simulink model "B52CostaTest"  (R2022a)
settings: Solver=VariableStepAuto  StartTime=0.0  StopTime=100  RelTol=1e-4  AbsTol=1e-4
values from neighbouring files (symbols this model uses):
  AinfK_h_B52 = -23    [B52.m]
  AinfK_p_B52 = 1.0    (= 1)    [B52.m]
  AinfK_s_B52 = 9.0    (= 9)    [B52.m]
  AinfNa_h_B52 = -37    [B52.m]
  AinfNa_p_B52 = 1.0    (= 1)    [B52.m]
  AinfNa_s_B52 = 5.0    (= 5)    [B52.m]
  AinfNarb_h_B52 = -61    [B52.m]    (also in CtrlParaSNSTuning.m)
  AinfNarb_p_B52 = 3    [B52.m]    (also in CtrlParaSNSTuning.m)
  AinfNarb_s_B52 = -1.0    (= -1)    [B52.m]    (also in CtrlParaSNSTuning.m)
  AK_B52_0 = 0.4    [B52.m]
  ANa_B52_0 = 0.4    [B52.m]
  ANarb_B52_0 = 0.1    [B52.m]    (also in CtrlParaSNSTuning.m; InitPara.m)
  BinfNa_h_B52 = -43.0    (= -43)    [B52.m]
  BinfNa_p_B52 = 1.0    (= 1)    [B52.m]
  BinfNa_s_B52 = 5.0    (= 5)    [B52.m]
  BNa_B52_0 = 0.4    [B52.m]
  Cm_B52 = 0.01    [B52.m]    (also in CtrlParaSNSTuning.m)
  EK_B52 = -70    [B52.m]
  EL_B52 = -62    [B52.m]    (also in CtrlParaSNSTuning.m)
  ENa_B52 = 30    [B52.m]
  ENarb_B52 = 30    [B52.m]    (also in CtrlParaSNSTuning.m)
  gK_B52 = 12    [B52.m]
  gL_B52 = 0.1    [B52.m]    (also in CtrlParaSNSTuning.m)
  gNa_B52 = 25    [B52.m]
  gNarb_B52 = 0.1    [B52.m]    (also in CtrlParaSNSTuning.m)
  pK_B52 = 4    [B52.m]
  pNa_B52 = 3    [B52.m]
  pNarb_B52 = 1    [B52.m]    (also in CtrlParaSNSTuning.m)
  RK_B52 = 0    [B52.m]
  RL_B52 = 0    [B52.m]    (also in CtrlParaSNSTuning.m)
  RNa_B52 = 0    [B52.m]
  RNarb_B52 = 0    [B52.m]    (also in CtrlParaSNSTuning.m)
  spikedur_B52 = 0.003    [B52.m]
  tAK_h_B52 = -8.0    (= -8)    [B52.m]
  tAK_p_B52 = 1.0    (= 1)    [B52.m]
  tAK_s_B52 = 10.0    (= 10)    [B52.m]
  tAK_tmax_B52 = 0.04    [B52.m]
  tAK_tmin_B52 = 0.004    [B52.m]
  tANa_h_B52 = -43    [B52.m]
  tANa_p_B52 = 1.0    (= 1)    [B52.m]
  tANa_s_B52 = 4.0    (= 4)    [B52.m]
  tANa_tmax_B52 = 0.006    [B52.m]
  tANa_tmin_B52 = 0.001    [B52.m]
  tANarb_h_B52 = -60    [B52.m]    (also in CtrlParaSNSTuning.m)
  tANarb_p_B52 = 1.0    (= 1)    [B52.m]    (also in CtrlParaSNSTuning.m)
  tANarb_s_B52 = 5    [B52.m]    (also in CtrlParaSNSTuning.m)
  tANarb_tmax_B52 = 20    [B52.m]    (also in CtrlParaSNSTuning.m)
  tANarb_tmin_B52 = 5    [B52.m]    (also in CtrlParaSNSTuning.m)
  tBNa_h_B52 = -38    [B52.m]
  tBNa_p_B52 = 1.0    (= 1)    [B52.m]
  tBNa_s_B52 = 10.0    (= 10)    [B52.m]
  tBNa_tmax_B52 = 0.02    [B52.m]
  tBNa_tmin_B52 = 0.005    [B52.m]
  V_B52_0 = -60    [B52.m]    (also in CtrlParaSNSTuning.m = -62; InitPara.m = -62)
undefined symbols (not defined in the file or in its folder): Iapp
libraries: simulink x1
settings Model: Creator=liyan  LastModifiedBy=liyan

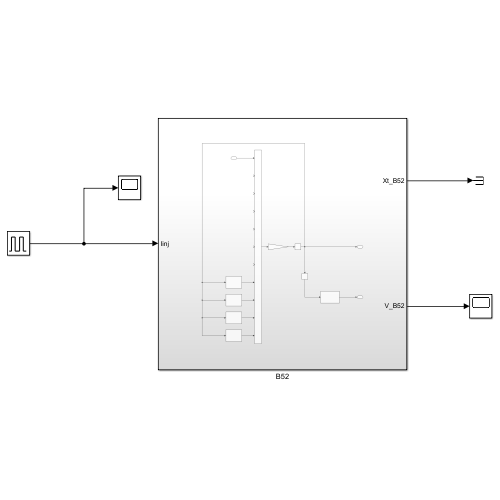
[thumbnail: Simulink's stored preview of the top-level diagram]
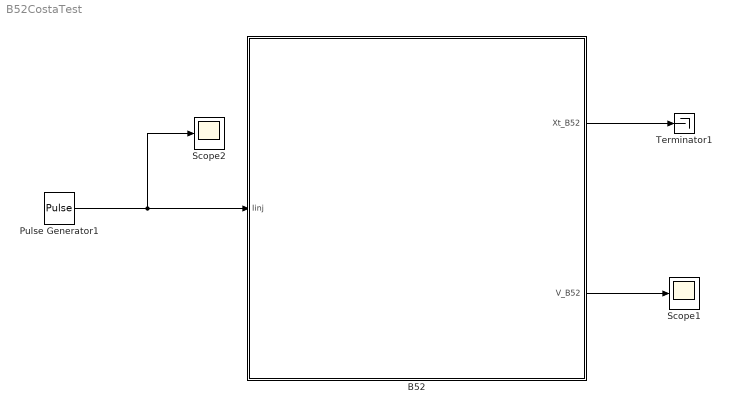
== system B52CostaTest ==
  B52 : Subsystem
  Pulse Generator1 : DiscretePulseGenerator  PulseType=Time based  Amplitude=Iapp  Period=100  PulseWidth=10/100*100  PhaseDelay=35
  Scope1 : Scope
  Scope2 : Scope
  Terminator1 : Terminator
  wires:
  Pulse Generator1/1 -> B52/1(Iinj), Scope2/1
  B52/2(Xt_B52) -> Terminator1/1
  B52/1(V_B52) -> Scope1/1

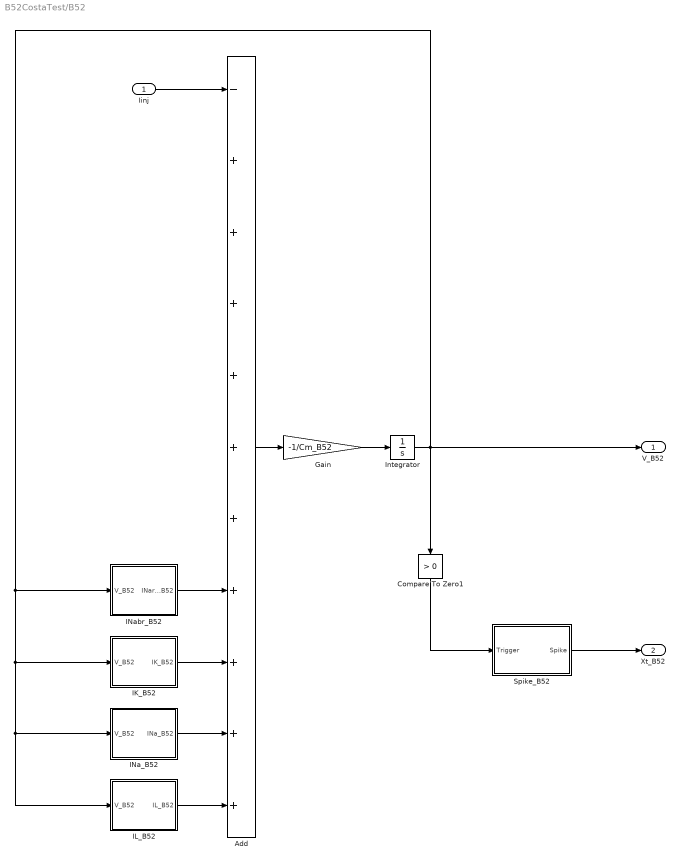
== system B52CostaTest/B52 ==
  Iinj : Inport
  Add : Sum  Inputs=-++++++++++
  Compare To Zero1 : simulink/Logic and Bit Operations/Compare To Zero  relop=>  OutDataTypeStr=boolean
  Gain : Gain  Gain=-1/Cm_B52
  IK_B52 : Subsystem
  IL_B52 : Subsystem
  INa_B52 : Subsystem
  INabr_B52 : Subsystem
  Integrator : Integrator  InitialCondition=V_B52_0
  Spike_B52 : Subsystem
  V_B52 : Outport
  Xt_B52 : Outport  Port=2
  wires:
  Gain/1 -> Integrator/1
  Add/1 -> Gain/1
  Compare To Zero1/1 -> Spike_B52/1(Trigger)
  INabr_B52/1(INarb_B52) -> Add/8
  Spike_B52/1(Spike) -> Xt_B52/1
  Integrator/1 -> V_B52/1, Compare To Zero1/1, INabr_B52/1(V_B52), IK_B52/1(V_B52), INa_B52/1(V_B52), IL_B52/1(V_B52)
  IL_B52/1(IL_B52) -> Add/11
  INa_B52/1(INa_B52) -> Add/10
  IK_B52/1(IK_B52) -> Add/9
  Iinj/1 -> Add/1

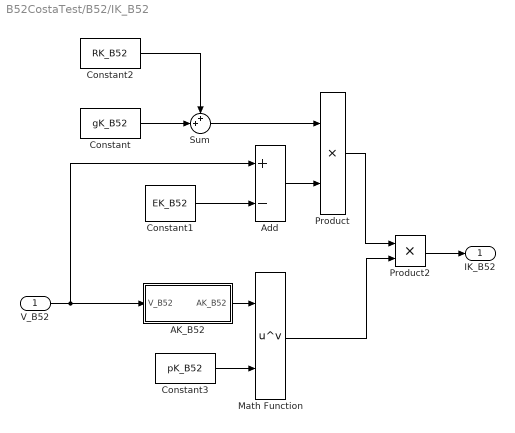
== system B52CostaTest/B52/IK_B52 ==
  V_B52 : Inport
  AK_B52 : Subsystem
  Add : Sum  Inputs=+-
  Constant : Constant  Value=gK_B52
  Constant1 : Constant  Value=EK_B52
  Constant2 : Constant  Value=RK_B52
  Constant3 : Constant  Value=pK_B52
  Math Function : Math  Operator=pow
  Product : Product
  Product2 : Product
  Sum : Sum  Inputs=++|
  IK_B52 : Outport
  wires:
  Add/1 -> Product/2
  Constant1/1 -> Add/2
  V_B52/1 -> AK_B52/1(V_B52), Add/1
  Product/1 -> Product2/1
  Math Function/1 -> Product2/2
  Product2/1 -> IK_B52/1
  Constant/1 -> Sum/2
  Sum/1 -> Product/1
  Constant2/1 -> Sum/1
  AK_B52/1(AK_B52) -> Math Function/1
  Constant3/1 -> Math Function/2

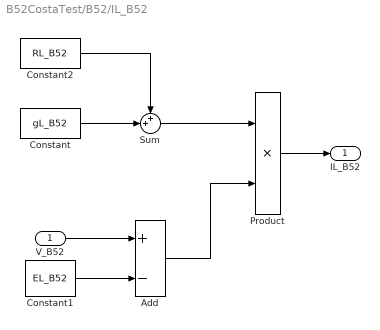
== system B52CostaTest/B52/IL_B52 ==
  V_B52 : Inport
  Add : Sum  Inputs=+-
  Constant : Constant  Value=gL_B52
  Constant1 : Constant  Value=EL_B52
  Constant2 : Constant  Value=RL_B52
  Product : Product
  Sum : Sum  Inputs=++|
  IL_B52 : Outport
  wires:
  Constant1/1 -> Add/2
  V_B52/1 -> Add/1
  Constant2/1 -> Sum/1
  Sum/1 -> Product/1
  Constant/1 -> Sum/2
  Add/1 -> Product/2
  Product/1 -> IL_B52/1

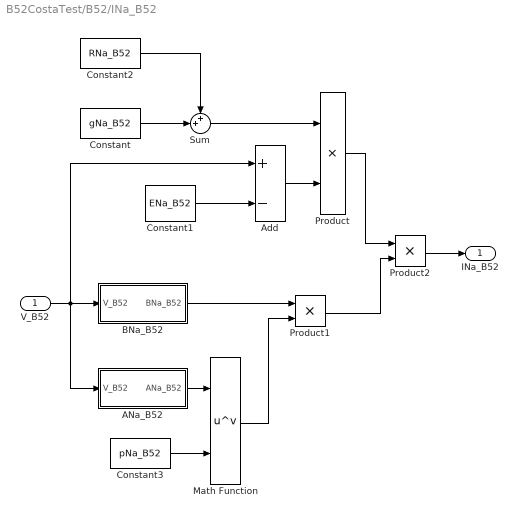
== system B52CostaTest/B52/INa_B52 ==
  V_B52 : Inport
  ANa_B52 : Subsystem
  Add : Sum  Inputs=+-
  BNa_B52 : Subsystem
  Constant : Constant  Value=gNa_B52
  Constant1 : Constant  Value=ENa_B52
  Constant2 : Constant  Value=RNa_B52
  Constant3 : Constant  Value=pNa_B52
  Math Function : Math  Operator=pow
  Product : Product
  Product1 : Product
  Product2 : Product
  Sum : Sum  Inputs=++|
  INa_B52 : Outport
  wires:
  Add/1 -> Product/2
  Constant1/1 -> Add/2
  V_B52/1 -> ANa_B52/1(V_B52), BNa_B52/1(V_B52), Add/1
  Product/1 -> Product2/1
  Product1/1 -> Product2/2
  Product2/1 -> INa_B52/1
  Constant/1 -> Sum/2
  Sum/1 -> Product/1
  Constant2/1 -> Sum/1
  ANa_B52/1(ANa_B52) -> Math Function/1
  Constant3/1 -> Math Function/2
  BNa_B52/1(BNa_B52) -> Product1/1
  Math Function/1 -> Product1/2

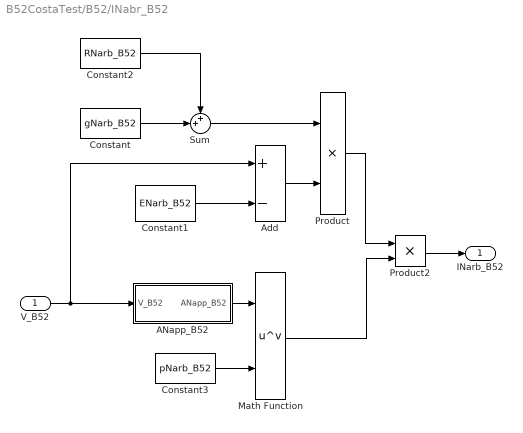
== system B52CostaTest/B52/INabr_B52 ==
  V_B52 : Inport
  ANapp_B52 : Subsystem
  Add : Sum  Inputs=+-
  Constant : Constant  Value=gNarb_B52
  Constant1 : Constant  Value=ENarb_B52
  Constant2 : Constant  Value=RNarb_B52
  Constant3 : Constant  Value=pNarb_B52
  Math Function : Math  Operator=pow
  Product : Product
  Product2 : Product
  Sum : Sum  Inputs=++|
  INarb_B52 : Outport
  wires:
  Add/1 -> Product/2
  Constant1/1 -> Add/2
  V_B52/1 -> ANapp_B52/1(V_B52), Add/1
  Product/1 -> Product2/1
  Math Function/1 -> Product2/2
  Product2/1 -> INarb_B52/1
  Constant/1 -> Sum/2
  Sum/1 -> Product/1
  Constant2/1 -> Sum/1
  ANapp_B52/1(ANapp_B52) -> Math Function/1
  Constant3/1 -> Math Function/2

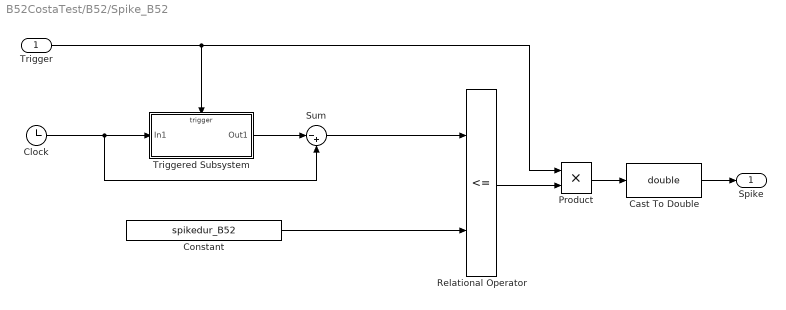
== system B52CostaTest/B52/Spike_B52 ==
  Trigger : Inport
  Cast To Double : DataTypeConversion  OutDataTypeStr=double  SaturateOnIntegerOverflow=off  RndMeth=Floor
  Clock : Clock
  Constant : Constant  Value=spikedur_B52
  Product : Product
  Relational Operator : RelationalOperator  Operator=<=  OutDataTypeStr=boolean  RndMeth=Simplest  InputSameDT=off
  Sum : Sum  Inputs=|-+
  Triggered Subsystem : Subsystem  TreatAsAtomicUnit=on
  Spike : Outport
  wires:
  Clock/1 -> Sum/2, Triggered Subsystem/1(In1)
  Triggered Subsystem/1(Out1) -> Sum/1
  Constant/1 -> Relational Operator/2
  Trigger/1 -> Triggered Subsystem/Trigger, Product/1
  Sum/1 -> Relational Operator/1
  Relational Operator/1 -> Product/2
  Product/1 -> Cast To Double/1
  Cast To Double/1 -> Spike/1

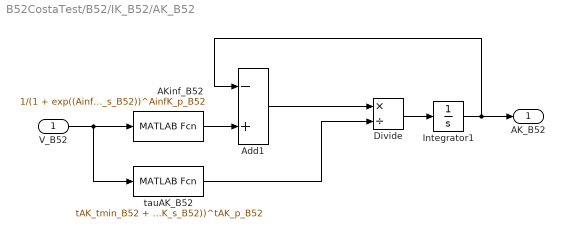
== system B52CostaTest/B52/IK_B52/AK_B52 ==
  V_B52 : Inport
  AKinf_B52 : MATLABFcn  MATLABFcn=1/(1 + exp((AinfK_h_B52 - u(1))/AinfK_s_B52))^AinfK_p_B52
  Add1 : Sum  Inputs=-+
  Divide : Product  Inputs=*/
  Integrator1 : Integrator  InitialCondition=AK_B52_0
  tauAK_B52 : MATLABFcn  MATLABFcn=tAK_tmin_B52 + (tAK_tmax_B52 - tAK_tmin_B52)/(1 + exp((u(1) - tAK_h_B52)/tAK_s_B52))^tAK_p_B52
  AK_B52 : Outport
  wires:
  tauAK_B52/1 -> Divide/2
  Divide/1 -> Integrator1/1
  V_B52/1 -> tauAK_B52/1, AKinf_B52/1
  Integrator1/1 -> Add1/1, AK_B52/1
  Add1/1 -> Divide/1
  AKinf_B52/1 -> Add1/2

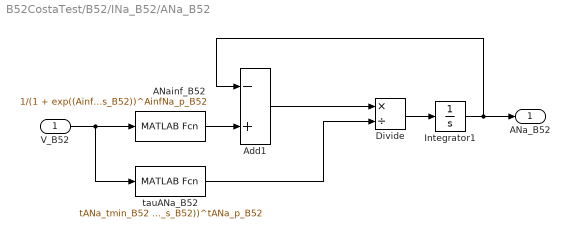
== system B52CostaTest/B52/INa_B52/ANa_B52 ==
  V_B52 : Inport
  ANainf_B52 : MATLABFcn  MATLABFcn=1/(1 + exp((AinfNa_h_B52 - u(1))/AinfNa_s_B52))^AinfNa_p_B52
  Add1 : Sum  Inputs=-+
  Divide : Product  Inputs=*/
  Integrator1 : Integrator  InitialCondition=ANa_B52_0
  tauANa_B52 : MATLABFcn  MATLABFcn=tANa_tmin_B52 + (tANa_tmax_B52 - tANa_tmin_B52)/(1 + exp((u(1) - tANa_h_B52)/tANa_s_B52))^tANa_p_B52
  ANa_B52 : Outport
  wires:
  tauANa_B52/1 -> Divide/2
  Divide/1 -> Integrator1/1
  V_B52/1 -> tauANa_B52/1, ANainf_B52/1
  Integrator1/1 -> Add1/1, ANa_B52/1
  Add1/1 -> Divide/1
  ANainf_B52/1 -> Add1/2

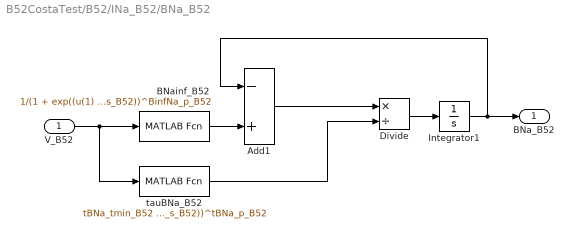
== system B52CostaTest/B52/INa_B52/BNa_B52 ==
  V_B52 : Inport
  Add1 : Sum  Inputs=-+
  BNainf_B52 : MATLABFcn  MATLABFcn=1/(1 + exp((u(1) - BinfNa_h_B52)/BinfNa_s_B52))^BinfNa_p_B52
  Divide : Product  Inputs=*/
  Integrator1 : Integrator  InitialCondition=BNa_B52_0
  tauBNa_B52 : MATLABFcn  MATLABFcn=tBNa_tmin_B52 + (tBNa_tmax_B52 - tBNa_tmin_B52)/(1 + exp((u(1) - tBNa_h_B52)/tBNa_s_B52))^tBNa_p_B52
  BNa_B52 : Outport
  wires:
  tauBNa_B52/1 -> Divide/2
  Divide/1 -> Integrator1/1
  V_B52/1 -> tauBNa_B52/1, BNainf_B52/1
  Integrator1/1 -> Add1/1, BNa_B52/1
  Add1/1 -> Divide/1
  BNainf_B52/1 -> Add1/2

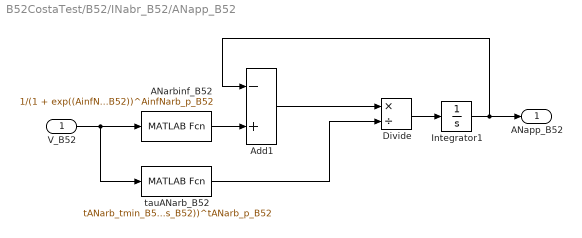
== system B52CostaTest/B52/INabr_B52/ANapp_B52 ==
  V_B52 : Inport
  ANarbinf_B52 : MATLABFcn  MATLABFcn=1/(1 + exp((AinfNarb_h_B52 - u(1))/AinfNarb_s_B52))^AinfNarb_p_B52
  Add1 : Sum  Inputs=-+
  Divide : Product  Inputs=*/
  Integrator1 : Integrator  InitialCondition=ANarb_B52_0
  tauANarb_B52 : MATLABFcn  MATLABFcn=tANarb_tmin_B52 + (tANarb_tmax_B52 - tANarb_tmin_B52)/(1 + exp((u(1) - tANarb_h_B52)/tANarb_s_B52))^tANarb_p_B52
  ANapp_B52 : Outport
  wires:
  tauANarb_B52/1 -> Divide/2
  Divide/1 -> Integrator1/1
  Integrator1/1 -> Add1/1, ANapp_B52/1
  Add1/1 -> Divide/1
  ANarbinf_B52/1 -> Add1/2
  V_B52/1 -> tauANarb_B52/1, ANarbinf_B52/1

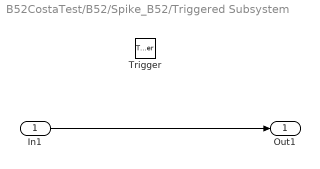
== system B52CostaTest/B52/Spike_B52/Triggered Subsystem ==
  In1 : Inport
  Trigger : TriggerPort  VariantControl=Variant
  Out1 : Outport
  wires:
  In1/1 -> Out1/1
